simulink model "sim_SoftwareIntheLoop_Compensator"  (R2015a)
settings: Solver=ode3  StartTime=0.0  StopTime=15  FixedStep=0.005  RelTol=1e-3
InitFcn:
  | % load parameters of the default quadrotor
  | disp('Quadrotor parameters loaded by InitFcn')
  | paramsFilters %load mdl_quadcopter as well!
  | 
  | % change to Simulation folder if in data folder
  | cd([matlabpath '/Simulation']);
undefined symbols (not defined in the file or in its folder): RSrun_sensorBiasRS, rt_yout, sampleTime_qcsim
settings Model: Creator=ra  LastModifiedBy=ra

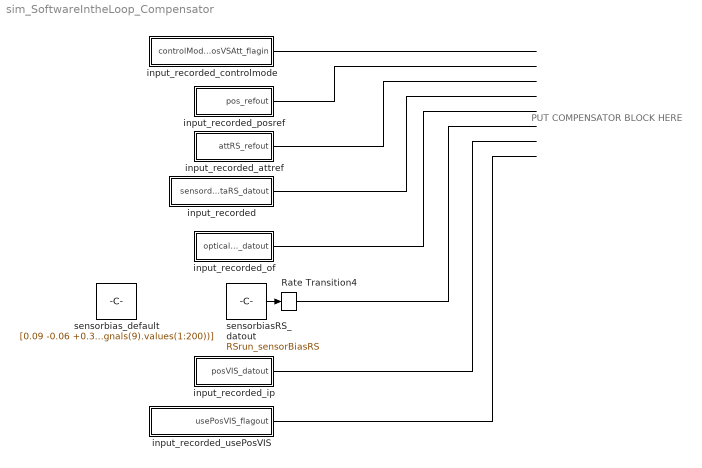
== system sim_SoftwareIntheLoop_Compensator ==
  note: PUT COMPENSATOR BLOCK HERE
  Rate Transition4 : RateTransition  OutPortSampleTime=sampleTime_qcsim
  input_recorded : Subsystem
  input_recorded_attref : Subsystem
  input_recorded_controlmode : Subsystem
  input_recorded_ip : Subsystem
  input_recorded_of : Subsystem
  input_recorded_posref : Subsystem
  input_recorded_usePosVIS : Subsystem
  sensorbiasRS_datout : Constant  Value=RSrun_sensorBiasRS
  sensorbias_default : Constant  Value=[0.09 -0.06 +0.337 -0.0095 -0.0075 0.0015 mean(rt_yout.signals(9).values(1:200))]
  wires:
  input_recorded_of/1(opticalFlowRS_datout) -> ?
  Rate Transition4/1 -> ?
  input_recorded/1(sensordataRS_datout) -> ?
  input_recorded_ip/1(posVIS_datout) -> ?
  input_recorded_attref/1(attRS_refout) -> ?
  input_recorded_posref/1(pos_refout) -> ?
  input_recorded_controlmode/1(controlModePosVSAtt_flagin) -> ?
  sensorbiasRS_datout/1 -> Rate Transition4/1
  input_recorded_usePosVIS/1(usePosVIS_flagout) -> ?

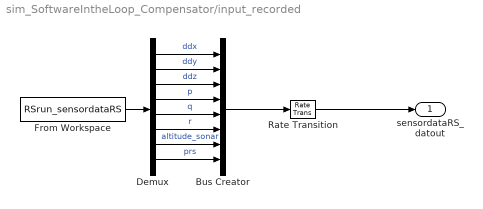
== system sim_SoftwareIntheLoop_Compensator/input_recorded ==
  Bus Creator : BusCreator  Inputs=8
  Demux : Demux  Outputs=8
  From Workspace : FromWorkspace  VariableName=RSrun_sensordataRS  SampleTime=sampleTime_qcsim
  Rate Transition : RateTransition  OutPortSampleTime=sampleTime_qcsim
  sensordataRS_datout : Outport
  wires:
  Demux/3 -> Bus Creator/3  "ddz"
  Demux/6 -> Bus Creator/6  "r"
  Demux/4 -> Bus Creator/4  "p"
  Demux/1 -> Bus Creator/1  "ddx"
  Demux/2 -> Bus Creator/2  "ddy"
  Bus Creator/1 -> Rate Transition/1
  Demux/5 -> Bus Creator/5  "q"
  From Workspace/1 -> Demux/1
  Demux/7 -> Bus Creator/7  "altitude_sonar"
  Rate Transition/1 -> sensordataRS_datout/1
  Demux/8 -> Bus Creator/8  "prs"

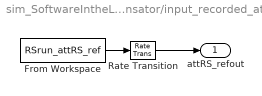
== system sim_SoftwareIntheLoop_Compensator/input_recorded_attref ==
  From Workspace : FromWorkspace  VariableName=RSrun_attRS_ref  SampleTime=sampleTime_qcsim
  Rate Transition : RateTransition  OutPortSampleTime=sampleTime_qcsim
  attRS_refout : Outport
  wires:
  From Workspace/1 -> Rate Transition/1
  Rate Transition/1 -> attRS_refout/1

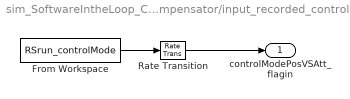
== system sim_SoftwareIntheLoop_Compensator/input_recorded_controlmode ==
  From Workspace : FromWorkspace  VariableName=RSrun_controlMode  SampleTime=sampleTime_qcsim
  Rate Transition : RateTransition  OutPortSampleTime=sampleTime_qcsim
  controlModePosVSAtt_flagin : Outport
  wires:
  From Workspace/1 -> Rate Transition/1
  Rate Transition/1 -> controlModePosVSAtt_flagin/1

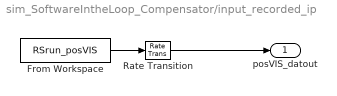
== system sim_SoftwareIntheLoop_Compensator/input_recorded_ip ==
  From Workspace : FromWorkspace  VariableName=RSrun_posVIS  SampleTime=sampleTime_qcsim
  Rate Transition : RateTransition  OutPortSampleTime=sampleTime_qcsim
  posVIS_datout : Outport
  wires:
  Rate Transition/1 -> posVIS_datout/1
  From Workspace/1 -> Rate Transition/1

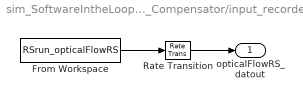
== system sim_SoftwareIntheLoop_Compensator/input_recorded_of ==
  From Workspace : FromWorkspace  VariableName=RSrun_opticalFlowRS  SampleTime=sampleTime_qcsim
  Rate Transition : RateTransition  OutPortSampleTime=sampleTime_qcsim
  opticalFlowRS_datout : Outport
  wires:
  Rate Transition/1 -> opticalFlowRS_datout/1
  From Workspace/1 -> Rate Transition/1

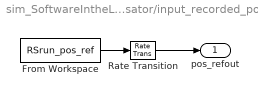
== system sim_SoftwareIntheLoop_Compensator/input_recorded_posref ==
  From Workspace : FromWorkspace  VariableName=RSrun_pos_ref  SampleTime=sampleTime_qcsim
  Rate Transition : RateTransition  OutPortSampleTime=sampleTime_qcsim
  pos_refout : Outport
  wires:
  Rate Transition/1 -> pos_refout/1
  From Workspace/1 -> Rate Transition/1

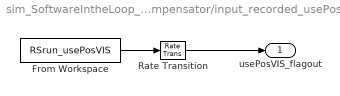
== system sim_SoftwareIntheLoop_Compensator/input_recorded_usePosVIS ==
  From Workspace : FromWorkspace  VariableName=RSrun_usePosVIS  SampleTime=sampleTime_qcsim
  Rate Transition : RateTransition  OutPortSampleTime=sampleTime_qcsim
  usePosVIS_flagout : Outport
  wires:
  From Workspace/1 -> Rate Transition/1
  Rate Transition/1 -> usePosVIS_flagout/1
